simulink model "MODELODETURBINADERIOV10"  (R2017b)
settings: Solver=ode1  StartTime=0.0  StopTime=1  FixedStep=Ts  MaxStep=1e-6  MinStep=1e-7  RelTol=1e-4  AbsTol=1e-3
values from neighbouring files (symbols this model uses):
  A = pi()*((D/2)^2)    [MODELOHIDRO.m]    (also in MODELOHIDROV10.m; MODELOHIDROV2.m; MODELOHIDROV3.m; MODELOHIDROV4.m)
  B = 0    [MODELOHIDRO.m]    (also in MODELOHIDROV10.m; MODELOHIDROV2.m; MODELOHIDROV3.m; MODELOHIDROV4.m)
  beta = 0    [MODELOHIDRO.m]    (also in MODELOHIDROV10.m; MODELOHIDROV2.m; MODELOHIDROV3.m; MODELOHIDROV4.m)
  Cinv = 10e-6    (= 1e-05)    [MODELOHIDROV10.m]    (also in MODELOHIDROV4.m; MODELOHIDROV7.m; MODELOHIDROV8.m = 3e-06)
  den = 1000    [MODELOHIDRO.m]    (also in MODELOHIDROV10.m; MODELOHIDROV2.m; MODELOHIDROV3.m; MODELOHIDROV4.m)
  J = 16.1919e-4    (= 0.00161919)    [MODELOHIDROV10.m]    (also in MODELOHIDROV2.m = 100; MODELOHIDROV3.m = 10; MODELOHIDROV4.m; MODELOHIDROV7.m)
  K1Ic = 100    [MODELOHIDROV10.m]    (also in MODELOHIDROV4.m; MODELOHIDROV7.m; MODELOHIDROV8.m; stateStadeInv.m)
  K1Vo = 50    [MODELOHIDROV10.m]    (also in MODELOHIDROV4.m; MODELOHIDROV7.m; MODELOHIDROV8.m; stateStadeInv.m)
  K2Ic = 5    [MODELOHIDROV10.m]    (also in MODELOHIDROV4.m; MODELOHIDROV7.m; MODELOHIDROV8.m; stateStadeInv.m)
  K2Vo = 0.5    [MODELOHIDROV10.m]    (also in MODELOHIDROV4.m; MODELOHIDROV7.m; MODELOHIDROV8.m; stateStadeInv.m)
  Kb = 1.8    [MODELOHIDRO.m]    (also in MODELOHIDROV10.m = 6.2; MODELOHIDROV2.m; MODELOHIDROV3.m; MODELOHIDROV4.m = 0.027)
  Kp = 0.4    [MODELOHIDRO.m]    (also in MODELOHIDROV10.m = 5.6627; MODELOHIDROV2.m; MODELOHIDROV3.m; MODELOHIDROV4.m = 0.027)
  Linv = 25e-3    (= 0.025)    [MODELOHIDROV10.m]    (also in MODELOHIDROV4.m; MODELOHIDROV7.m; MODELOHIDROV8.m = 0.02345)
  r = D/2    (= 0.5)    [MODELOHIDRO.m]    (also in MODELOHIDROV10.m; MODELOHIDROV2.m; MODELOHIDROV3.m; MODELOHIDROV4.m)
  Ri = 0.6    [MODELOHIDRO.m]    (also in MODELOHIDROV10.m = 0.973; MODELOHIDROV2.m; MODELOHIDROV3.m; MODELOHIDROV4.m = 1)
  T_d = 0    [MODELOHIDRO.m]    (also in MODELOHIDROV10.m; MODELOHIDROV2.m; MODELOHIDROV3.m; MODELOHIDROV4.m)
  Vg = 150    [MODELOHIDROV10.m]    (also in MODELOHIDROV4.m; MODELOHIDROV7.m; MODELOHIDROV8.m)
undefined symbols (not defined in the file or in its folder): sigbuilder_block
libraries: powerlib_extras x3, simulink x2, powerlib_meascontrol x1
settings Model: ExtModeTrigMode=oneshot  ExtModeArmWhenConnect=off  ExtModeAutoUpdateStatusClock=off  Creator=Giroux/Sybille  LastModifiedBy=Hp 14
settings DataIOCC: SaveFinalState=on  SaveFormat=Structure  SignalLoggingSaveFormat=ModelDataLogs  SaveOutput=off  SaveTime=off  SignalLoggingName=sigsOut
settings OptimizationCC: BlockReduction=off  BooleanDataType=off  ExpressionDepthLimit=2147483647  InitFltsAndDblsToZero=on  LifeSpan=inf  BufferReusableBoundary=off
settings DebuggingCC: UnderspecifiedInitializationDetection=Classic  MergeDetectMultiDrivingBlocksExec=none  CheckExecutionContextPreStartOutputMsg=on  CheckExecutionContextRuntimeOutputMsg=on  SignalResolutionControl=TryResolveAllWithWarning  MultiTaskDSMMsg=warning  MultiTaskCondExecSysMsg=none  FcnCallInpInsideContextMsg=warning  UnconnectedLineMsg=none  BusObjectLabelMismatch=none  StateNameClashWarn=warning  SFUnexpectedBacktrackingDiag=warning  SFNoUnconditionalDefaultTransitionDiag=warning  SFExecutionAtInitializationDiag=none
settings HardwareCC: ProdBitPerPointer=32  ProdBitPerSizeT=32  ProdBitPerPtrDiffT=32  ProdLargestAtomicFloat=None  ProdIntDivRoundTo=Undefined  ProdEndianess=Unspecified  ProdWordSize=32  ProdHWDeviceType=32-bit Generic  TargetBitPerPointer=64  TargetBitPerSizeT=64  TargetBitPerPtrDiffT=64  TargetLongLongMode=on  TargetIntDivRoundTo=Zero  TargetEndianess=LittleEndian  TargetWordSize=64  TargetHWDeviceType=MATLAB Host  ProdEqTarget=off
settings ModelReferenceCC: PropagateSignalLabelsOutOfModel=off
settings CodeAppCC: StateflowObjectComments=on
settings GRTTargetCC: TargetLangStandard=C89/C90 (ANSI)  GeneratePreprocessorConditionals=Disable all  CombineOutputUpdateFcns=off  GRTInterface=on
settings ConfigComp: CovMetricSettings=dw  CovHtmlReporting=on  CovSaveCumulativeToWorkspaceVar=on  CovSaveSingleToWorkspaceVar=on  CovExternalEMLEnable=off
settings SimscapeCC: SimscapeNormalizeSystem=off

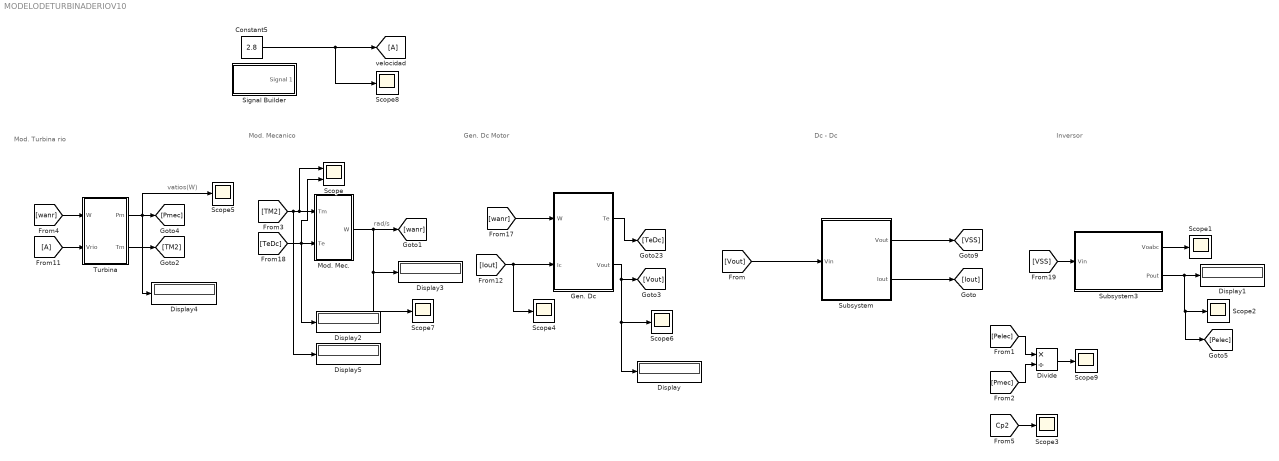
== system MODELODETURBINADERIOV10 ==
  note: vatios(W)
  note: rad/s
  note: Mod. Mecanico
  note: Gen. Dc Motor
  note: Mod. Turbina rio
  note: Inversor
  note: Dc - Dc
  Constant5 : Constant  Value=2.8
  Display{,1..5} (6 alike) : Display
  Divide : Product  Inputs=*/
  Gen. Dc : Subsystem
  Mod. Mec. : Subsystem
  Scope : Scope  NumInputPorts=2
  Scope{1..9} (9 alike) : Scope
  Signal Builder : Subsystem  Tag=STV Subsys  LoadFcn=sigbuilder_block('load');  StartFcn=sigbuilder_block('start');  StopFcn=sigbuilder_block('stop');  ClipboardFcn=sigbuilder_block('clipboard');  mask(Sigbuilder block){tuvar=[0:10]}
      mask help: Simulink:masks:SigbuilderBlock_MD
      mask init:
      | if ~strcmp(get_param(bdroot(gcbh),'SimulationStatus'),'stopped') tuvar = sigbuilder_block('maskInit'); end
      settings: CopyFcn=sigbuilder_block('copy');  DeleteFcn=sigbuilder_block('delete');  ModelCloseFcn=sigbuilder_block('modelClose');  PreSaveFcn=sigbuilder_block('preSave');  PauseFcn=sigbuilder_block('pause');  ContinueFcn=sigbuilder_block('continue');  NameChangeFcn=sigbuilder_block('namechange');  OpenFcn=sigbuilder_block('open',[437.25 153 550.5 359.25 ]);  CloseFcn=sigbuilder_block('close');
      mask Display: plot(0, 0, 100, 100,[2, 2, 32, 32, 2], [68, 8, 8, 68, 68],[32, 2], [38, 38], [32, 19, 2],[53, 60, 44], [32, 17, 17, 2],[16, 16, 31, 31]);txt = getActiveGroup(gcbh);text(2, 100, txt,'verticalAlignment', 'top');
  Subsystem : Subsystem
  Subsystem3 : Subsystem
  Turbina : Subsystem
  wires:
  [wanr] -> Gen. Dc/1(W)
  [TM2] -> Scope/1, Mod. Mec./1(Tm), Display5/1
  [wanr] -> Turbina/1(W)
  [TeDc] -> Display2/1, Scope/2, Mod. Mec./2(Te)
  Gen. Dc/1(Te) -> [TeDc]
  Turbina/1(Pm) -> [Pmec], Scope5/1, Display4/1
  Gen. Dc/2(Vout) -> [Vout], Scope6/1, Display/1
  Turbina/2(Tm) -> [TM2]
  [A] -> Turbina/2(Vrio)
  [Iout] -> Scope4/1, Gen. Dc/2(Ic)
  [VSS] -> Subsystem3/1(Vin)
  Subsystem3/1("Voabc ") -> Scope1/1
  Subsystem/1(Vout) -> [VSS]
  Subsystem/2(Iout) -> [Iout]
  [Vout] -> Subsystem/1(Vin)
  Subsystem3/2(Pout) -> Scope2/1, [Pelec], Display1/1
  [Pelec] -> Divide/1
  [Pmec] -> Divide/2
  Divide/1 -> Scope9/1
  [Cp2] -> Scope3/1
  Mod. Mec./1(W) -> Scope7/1, Display3/1, [wanr]
  Constant5/1 -> [A], Scope8/1

== system MODELODETURBINADERIOV10/Gen. Dc ==
  note: Calculo del par electrico con la corriente en la carga
  note: Se emplean parametro de un motor dc para 18.5Kw debido a que fueron con los que mejor trabajo
  W : Inport
  Ic : Inport  Port=2
  Motor iman. : Subsystem
  Par elec. : Subsystem
  Te : Outport
  Vout : Outport  Port=2
  wires:
  Motor iman./1(Out1) -> Vout/1
  Par elec./1(Te) -> Te/1
  W/1 -> Motor iman./2(W)
  Ic/1 -> Par elec./1(Ic), Motor iman./1(I)

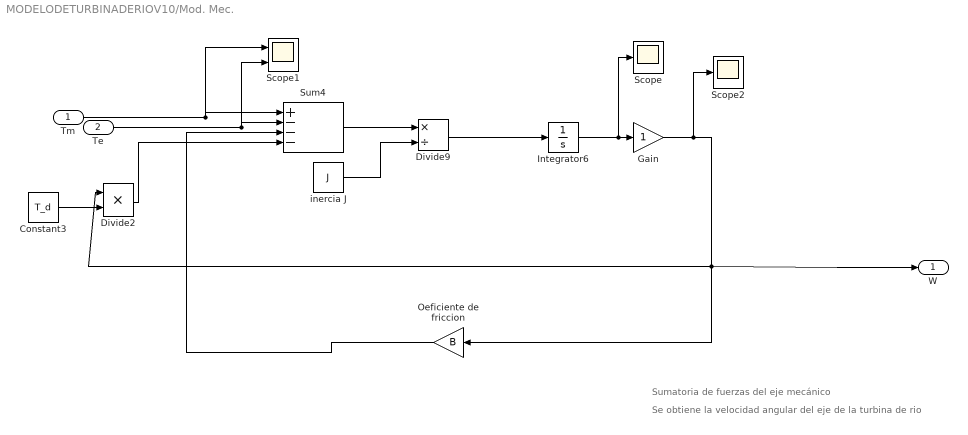
== system MODELODETURBINADERIOV10/Mod. Mec. ==
  note: Se obtiene la velocidad angular del eje de la turbina de rio
  note: Sumatoria de fuerzas del eje mecánico
  Tm : Inport
  Te : Inport  Port=2
  Constant3 : Constant  Value=T_d
  Divide2 : Product  Inputs=**
  Divide9 : Product  Inputs=*/
  Gain : Gain
  Integrator6 : Integrator  InitialCondition=10
  Oeficiente de friccion : Gain  Gain=B
  Scope : Scope
  Scope1 : Scope  NumInputPorts=2
  Scope2 : Scope
  Sum4 : Sum  Inputs=|+---
  inercia J : Constant  Value=J
  W : Outport
  wires:
  inercia J/1 -> Divide9/2
  Constant3/1 -> Divide2/2
  Divide2/1 -> Sum4/4
  Oeficiente de friccion/1 -> Sum4/3
  Sum4/1 -> Divide9/1
  Tm/1 -> Scope1/1, Sum4/1
  Te/1 -> Scope1/2, Sum4/2
  Divide9/1 -> Integrator6/1
  Integrator6/1 -> Scope/1, Gain/1
  Gain/1 -> Scope2/1, Oeficiente de friccion/1, W/1, Divide2/1

== system MODELODETURBINADERIOV10/Signal Builder ==
  Demux : Demux  Tag=STV Demux  Outputs=1
  FromWs : FromWorkspace  Tag=STV FromWs  VariableName=tuvar  SampleTime=0
      SigBuilderData=|
      | common.afterFinalStr = 'Extrapolate'
      | common.sampleTime = 0
      | dataSet.timeRange = [0 1]
      | dataSet.name = 'Group 1'
      | sbobj.Groups.Name = 'Group 1'
      | sbobj.Groups.Signals.Name = 'Signal 1'
      | sbobj.Groups.Signals.XData = [0 0.32 0.32 1]
      | sbobj.Groups.Signals.YData = [2.6 2.6 2.8 2.8]
      | sbobj.Groups.TimeRange = [0 1]
  Signal 1 : Outport  Tag=STV Outport
  wires:
  Demux/1 -> Signal 1/1
  FromWs/1 -> Demux/1

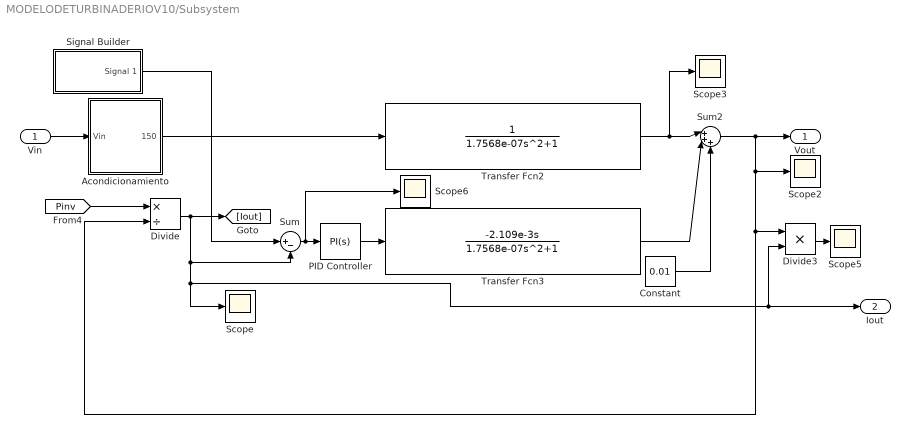
== system MODELODETURBINADERIOV10/Subsystem ==
  Vin : Inport
  Acondicionamiento : Subsystem
  Constant : Constant  Value=0.01
  Divide : Product  Inputs=*/
  Divide3 : Product  Inputs=**
  PID Controller : simulink/Continuous/PID Controller  Controller=PI  TimeDomain=Continuous-time  SampleTime=-1  IntegratorMethod=Forward Euler  FilterMethod=Forward Euler  Form=Parallel  UseFilter=on  ControllerParametersSource=internal  P=30  I=55  D=0  N=100  InitialConditionSource=internal  InitialConditionForIntegrator=0  InitialConditionForFilter=0  ExternalReset=none  LimitOutput=off  UpperSaturationLimit=inf  LowerSaturationLimit=-inf  LinearizeAsGain=on  AntiWindupMode=none  Kb=1  TrackingMode=off  Kt=1  PParamMin=[]  PParamMax=[]  IParamMin=[]  IParamMax=[]  DParamMin=[]  DParamMax=[]  NParamMin=[]  NParamMax=[]  KbParamMin=[]  KbParamMax=[]  KtParamMin=[]  KtParamMax=[]  POutMin=[]  POutMax=[]  IOutMin=[]  IOutMax=[]  DOutMin=[]  DOutMax=[]  NOutMin=[]  NOutMax=[]  KbOutMin=[]  KbOutMax=[]  KtOutMin=[]  KtOutMax=[]  IntegratorOutMin=[]  IntegratorOutMax=[]  FilterOutMin=[]  FilterOutMax=[]  SumOutMin=[]  SumOutMax=[]  SumI1OutMin=[]  SumI1OutMax=[]  SumI2OutMin=[]  SumI2OutMax=[]  SumI3OutMin=[]  SumI3OutMax=[]  SumDOutMin=[]  SumDOutMax=[]  SaturationOutMin=[]  SaturationOutMax=[]  IntegratorContinuousStateAttributes=''  IntegratorStateMustResolveToSignalObject=off  IntegratorRTWStateStorageClass=Auto  FilterContinuousStateAttributes=''  FilterStateMustResolveToSignalObject=off  FilterRTWStateStorageClass=Auto  DifferentiatorICPrevScaledInput=0  DifferentiatorOutMin=[]  DifferentiatorOutMax=[]  InitialConditionSetting=State (most efficient)  FilterDiffOutCoefMin=[]  FilterDiffOutCoefMax=[]  SumDenOutMin=[]  SumDenOutMax=[]  SumNumOutMin=[]  SumNumOutMax=[]  ReciprocalOutMin=[]  ReciprocalOutMax=[]  DivideOutMin=[]  DivideOutMax=[]  TunerSelectOption=Transfer Function Based (PID Tuner App)
  Scope{,2..3,5..6} (5 alike) : Scope
  Signal Builder : Subsystem  Tag=STV Subsys  LoadFcn=sigbuilder_block('load');  StartFcn=sigbuilder_block('start');  StopFcn=sigbuilder_block('stop');  ClipboardFcn=sigbuilder_block('clipboard');  mask(Sigbuilder block){tuvar=[0:10]}
      mask help: Simulink:masks:SigbuilderBlock_MD
      mask init:
      | if ~strcmp(get_param(bdroot(gcbh),'SimulationStatus'),'stopped') tuvar = sigbuilder_block('maskInit'); end
      settings: CopyFcn=sigbuilder_block('copy');  DeleteFcn=sigbuilder_block('delete');  ModelCloseFcn=sigbuilder_block('modelClose');  PreSaveFcn=sigbuilder_block('preSave');  PauseFcn=sigbuilder_block('pause');  ContinueFcn=sigbuilder_block('continue');  NameChangeFcn=sigbuilder_block('namechange');  OpenFcn=sigbuilder_block('open',[437.25 153 550.5 359.25 ]);  CloseFcn=sigbuilder_block('close');
      mask Display: plot(0, 0, 100, 100,[2, 2, 32, 32, 2], [68, 8, 8, 68, 68],[32, 2], [38, 38], [32, 19, 2],[53, 60, 44], [32, 17, 17, 2],[16, 16, 31, 31]);txt = getActiveGroup(gcbh);text(2, 100, txt,'verticalAlignment', 'top');
  Sum : Sum  Inputs=|+-
  Sum2 : Sum  Inputs=|+++
  Transfer Fcn2 : TransferFcn  Denominator=[1.7568e-07 0 1]
  Transfer Fcn3 : TransferFcn  Numerator=[-2.109e-3 0]  Denominator=[1.7568e-07 0 1]
  Vout : Outport
  Iout : Outport  Port=2
  wires:
  Transfer Fcn3/1 -> Sum2/2
  Transfer Fcn2/1 -> Scope3/1, Sum2/1
  Vin/1 -> Acondicionamiento/1(Vin)
  [Pinv] -> Divide/1
  Divide/1 -> Sum/2, Divide3/2, Iout/1, Scope/1, [Iout]
  Constant/1 -> Sum2/3
  Sum2/1 -> Divide/2, Divide3/1, Scope2/1, Vout/1
  Divide3/1 -> Scope5/1
  Acondicionamiento/1(150) -> Transfer Fcn2/1
  PID Controller/1 -> Transfer Fcn3/1
  Sum/1 -> Scope6/1, PID Controller/1
  Signal Builder/1(Signal 1) -> Sum/1

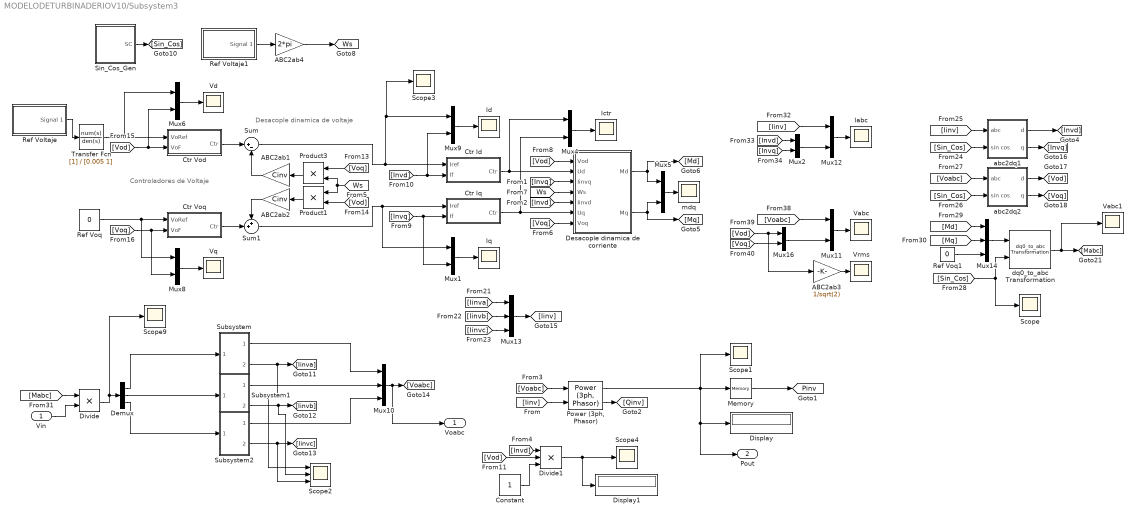
== system MODELODETURBINADERIOV10/Subsystem3 ==
  note: Desacople dinamica de voltaje
  note: Controladores de Voltaje
  Vin : Inport
  ABC2ab1 : Gain  Gain=Cinv  SaturateOnIntegerOverflow=on  OutDataTypeStr=Inherit: Same as input  ParamDataTypeStr=Inherit: Same as input
  ABC2ab2 : Gain  Gain=Cinv  SaturateOnIntegerOverflow=on  OutDataTypeStr=Inherit: Same as input  ParamDataTypeStr=Inherit: Same as input
  ABC2ab3 : Gain  Gain=1/sqrt(2)  SaturateOnIntegerOverflow=on  OutDataTypeStr=Inherit: Same as input  ParamDataTypeStr=Inherit: Same as input
  ABC2ab4 : Gain  Gain=2*pi  SaturateOnIntegerOverflow=on  OutDataTypeStr=Inherit: Same as input  ParamDataTypeStr=Inherit: Same as input
  Constant : Constant
  Ctr Id : Subsystem
  Ctr Iq : Subsystem
  Ctr Vod : Subsystem
  Ctr Voq : Subsystem
  Demux : Demux  Outputs=3
  Desacople dinamica de corriente : Subsystem
  Display : Display
  Display1 : Display
  Divide : Product  Inputs=**
  Divide1 : Product  Inputs=***
  Iabc : Scope
  Ictr : Scope
  Id : Scope
  Iq : Scope
  Memory : Memory
  Mux{1..2,4..6,8..9,11..12,16} (10 alike) : Mux  Inputs=2
  Mux10 : Mux  Inputs=3
  Mux13 : Mux  Inputs=3
  Mux14 : Mux  Inputs=3
  "Power (3ph, Phasor)" : powerlib_meascontrol/Measurements/Power (3ph, Phasor)
      settings: SourceProductName=Simscape Power Systems  SourceProductBaseCode=PS
  Product1 : Product  OutDataTypeStr=double  RndMeth=Zero
  Product3 : Product  OutDataTypeStr=double  RndMeth=Zero
  Ref Voltaje : Subsystem  Tag=STV Subsys  LoadFcn=sigbuilder_block('load');  StartFcn=sigbuilder_block('start');  StopFcn=sigbuilder_block('stop');  ClipboardFcn=sigbuilder_block('clipboard');  mask(Sigbuilder block){tuvar=[0:10]}
      mask help: Sigbuilder GUI
      mask init:
      | if ~strcmp(get_param(bdroot(gcbh),'SimulationStatus'),'stopped') tuvar = sigbuilder_block('maskInit'); end
      settings: CopyFcn=sigbuilder_block('copy');  DeleteFcn=sigbuilder_block('delete');  ModelCloseFcn=sigbuilder_block('modelClose');  PreSaveFcn=sigbuilder_block('preSave');  PauseFcn=sigbuilder_block('pause')  ContinueFcn=sigbuilder_block('continue')  NameChangeFcn=sigbuilder_block('namechange');  OpenFcn=sigbuilder_block('open',[437.25 117 550.5 399 ]);  CloseFcn=sigbuilder_block('close');
      mask Display: plot(0, 0, 100, 100,[2, 2, 32, 32, 2], [68, 8, 8, 68, 68],[32, 2], [38, 38], [32, 19, 2],[53, 60, 44], [32, 17, 17, 2],[16, 16, 31, 31]);txt = getActiveGroup(gcbh);text(2, 100, txt,'verticalAlignment', 'top');
  Ref Voltaje1 : Subsystem  Tag=STV Subsys  LoadFcn=sigbuilder_block('load');  StartFcn=sigbuilder_block('start');  StopFcn=sigbuilder_block('stop');  ClipboardFcn=sigbuilder_block('clipboard');  mask(Sigbuilder block){tuvar=[0:10]}
      mask help: Sigbuilder GUI
      mask init:
      | if ~strcmp(get_param(bdroot(gcbh),'SimulationStatus'),'stopped') tuvar = sigbuilder_block('maskInit'); end
      settings: CopyFcn=sigbuilder_block('copy');  DeleteFcn=sigbuilder_block('delete');  ModelCloseFcn=sigbuilder_block('modelClose');  PreSaveFcn=sigbuilder_block('preSave');  PauseFcn=sigbuilder_block('pause')  ContinueFcn=sigbuilder_block('continue')  NameChangeFcn=sigbuilder_block('namechange');  OpenFcn=sigbuilder_block('open',[437.25 117 550.5 399 ]);  CloseFcn=sigbuilder_block('close');
      mask Display: plot(0, 0, 100, 100,[2, 2, 32, 32, 2], [68, 8, 8, 68, 68],[32, 2], [38, 38], [32, 19, 2],[53, 60, 44], [32, 17, 17, 2],[16, 16, 31, 31]);txt = getActiveGroup(gcbh);text(2, 100, txt,'verticalAlignment', 'top');
  Ref Voq : Constant  Value=0
  Ref Voq1 : Constant  Value=0
  Scope{,1,3..4,9} (5 alike) : Scope
  Scope2 : Scope  NumInputPorts=3
  Sin_Cos_Gen : Subsystem
  Subsystem : Subsystem
  Subsystem1 : Subsystem
  Subsystem2 : Subsystem
  Sum : Sum  Inputs=|+-
  Sum1 : Sum  Inputs=++|
  Transfer Fcn : TransferFcn  Denominator=[0.005 1]
  Vabc : Scope
  Vabc1 : Scope
  Vd : Scope
  Vq : Scope
  Vrms : Scope
  abc2dq1 : Subsystem
  abc2dq2 : Subsystem
  dq0_to_abc Transformation : powerlib_extras/Measurements/dq0_to_abc Transformation
  mdq : Scope
  "Voabc " : Outport
  Pout : Outport  Port=2
  tag scope: Pinv=global, Ws=global
  wires:
  Demux/2 -> Subsystem1/1(Vin)
  Subsystem2/2(Iout) -> Scope2/3, [Iinvc]
  Subsystem1/1(Vout) -> Mux10/2
  Subsystem/2(Iout) -> Scope2/1, [Iinva]
  Mux9/1 -> Id/1
  [Vod] -> Desacople dinamica de corriente/1(Vod)
  Ctr Id/1(Ctr) -> Desacople dinamica de corriente/2(Ud), Mux4/1
  [Invd] -> Desacople dinamica de corriente/5(Iinvd)
  [Invq] -> Desacople dinamica de corriente/3(Iinvq)
  Mux4/1 -> Ictr/1
  Mux5/1 -> mdq/1
  Product1/1 -> ABC2ab2/1
  [Invq] -> Ctr Iq/2(If), Mux1/2
  [Invd] -> Ctr Id/2(If), Mux9/2
  [Voq] -> Desacople dinamica de corriente/7(Voq)
  ABC2ab4/1 -> [Ws]
  [Ws] -> Desacople dinamica de corriente/4(Ws)
  Sum1/1 -> Ctr Iq/1(Iref), Mux1/1
  Ctr Iq/1(Ctr) -> Desacople dinamica de corriente/6(Uq), Mux4/2
  Mux1/1 -> Iq/1
  [Ws] -> Product3/2, Product1/1
  Sum/1 -> Ctr Id/1(Iref), Scope3/1, Mux9/1
  ABC2ab1/1 -> Sum/2
  Product3/1 -> ABC2ab1/1
  [Voq] -> Product3/1
  Mux6/1 -> Vd/1
  [Vod] -> Mux6/2, Ctr Vod/2(VoF)
  Ctr Voq/1(Ctr) -> Sum1/2
  ABC2ab2/1 -> Sum1/1
  [Vod] -> Product1/2
  Ctr Vod/1(Ctr) -> Sum/1
  Ref Voq/1 -> Mux8/1, Ctr Voq/1(VoRef)
  Ref Voltaje/1(Signal 1) -> Transfer Fcn/1
  [Voq] -> Mux8/2, Ctr Voq/2(VoF)
  Mux8/1 -> Vq/1
  [Iinva] -> Mux13/1
  Mux13/1 -> [Iinv]
  Mux12/1 -> Iabc/1
  [Iinv] -> abc2dq1/1(abc)
  [Iinvb] -> Mux13/2
  [Sin_Cos] -> abc2dq1/2(sin cos)
  Mux11/1 -> Vabc/1
  [Iinvc] -> Mux13/3
  [Iinv] -> Mux12/1
  [Voabc] -> abc2dq2/1(abc)
  [Vod] -> Mux16/1, ABC2ab3/1
  ABC2ab3/1 -> Vrms/1
  Sin_Cos_Gen/1(SC) -> [Sin_Cos]
  Ref Voq1/1 -> Mux14/3
  [Md] -> Mux14/1
  Desacople dinamica de corriente/2(Mq) -> Mux5/2, [Mq]
  abc2dq2/2(q) -> [Voq]
  [Sin_Cos] -> abc2dq2/2(sin cos)
  [Mq] -> Mux14/2
  dq0_to_abc Transformation/1 -> [Mabc], Vabc1/1
  abc2dq1/2(q) -> [Invq]
  abc2dq2/1(d) -> [Vod]
  [Sin_Cos] -> Scope/1, dq0_to_abc Transformation/2
  [Invd] -> Mux2/1
  Desacople dinamica de corriente/1(Md) -> Mux5/1, [Md]
  [Voabc] -> Mux11/1
  Mux2/1 -> Mux12/2
  [Invq] -> Mux2/2
  [Voq] -> Mux16/2
  Mux16/1 -> Mux11/2
  Mux14/1 -> dq0_to_abc Transformation/1
  Ref Voltaje1/1(Signal 1) -> ABC2ab4/1
  Transfer Fcn/1 -> Mux6/1, Ctr Vod/1(VoRef)
  Subsystem/1(Vout) -> Mux10/1
  Demux/3 -> Subsystem2/1(Vin)
  Demux/1 -> Subsystem/1(Vin)
  Mux10/1 -> "Voabc "/1, [Voabc]
  Subsystem1/2(Iout) -> Scope2/2, [Iinvb]
  [Mabc] -> Divide/1
  Divide/1 -> Scope9/1, Demux/1
  Subsystem2/1(Vout) -> Mux10/3
  [Iinv] -> "Power (3ph, Phasor)"/2
  [Voabc] -> "Power (3ph, Phasor)"/1
  "Power (3ph, Phasor)"/1 -> Pout/1, Display/1, Scope1/1, Memory/1
  "Power (3ph, Phasor)"/2 -> [Qinv]
  Memory/1 -> [Pinv]
  Vin/1 -> Divide/2
  abc2dq1/1(d) -> [Invd]
  Constant/1 -> Divide1/3
  [Invd] -> Divide1/1
  [Vod] -> Divide1/2
  Divide1/1 -> Display1/1, Scope4/1

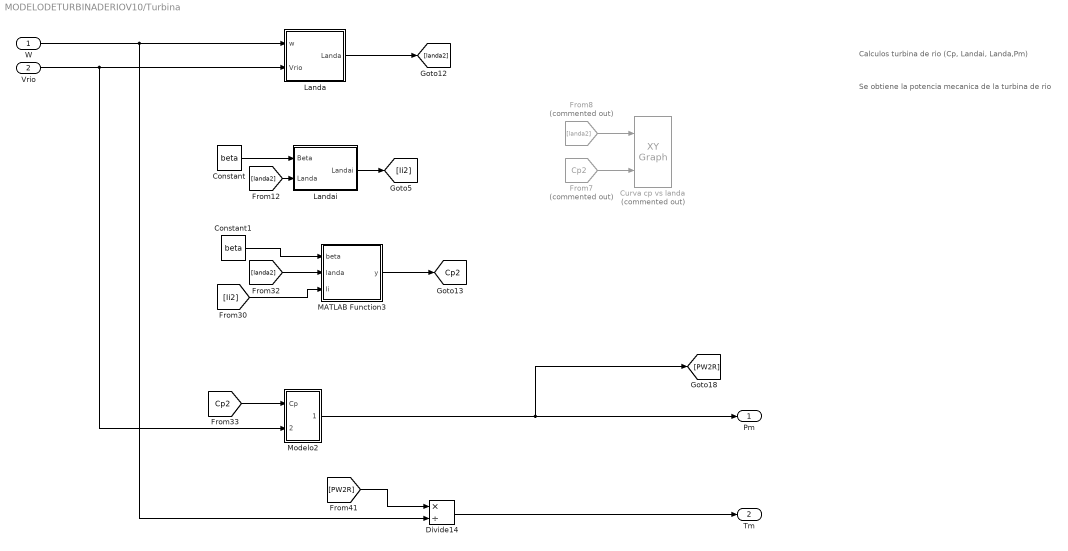
== system MODELODETURBINADERIOV10/Turbina ==
  note: Calculos turbina de rio (Cp, Landai, Landa,Pm)
  note: Se obtiene la potencia mecanica de la turbina de rio
  W : Inport
  Vrio : Inport  Port=2
  Constant : Constant  Value=beta
  Constant1 : Constant  Value=beta
  Curva cp vs landa : simulink/Sinks/XY Graph  Commented=on  xmin=1  xmax=20  ymin=0  ymax=0.56  st=0.1
  Divide14 : Product  Inputs=*/
  From7 : From  Commented=on  GotoTag=Cp2
  From8 : From  Commented=on  GotoTag=landa2
  Landa : Subsystem
  Landai : Subsystem
  MATLAB Function3 : MATLAB Function  TreatAsAtomicUnit=on
  Modelo2 : Subsystem
  Pm : Outport
  Tm : Outport  Port=2
  tag scope: Cp2=global
  wires:
  Constant1/1 -> MATLAB Function3/1(beta)
  Divide14/1 -> Tm/1
  [Ii2] -> MATLAB Function3/3(Ii)
  [Cp2] -> Modelo2/1(Cp)
  [PW2R] -> Divide14/1
  W/1 -> Divide14/2, Landa/1(w)
  [landa2] -> MATLAB Function3/2(landa)
  Vrio/1 -> Modelo2/2(Vrio), Landa/2(Vrio)
  Landa/1(Landa) -> [landa2]
  MATLAB Function3/1(y) -> [Cp2]
  From8/1 -> Curva cp vs landa/1
  Constant/1 -> Landai/1(Beta)
  [landa2] -> Landai/2(Landa)
  Modelo2/1(Pm) -> [PW2R], Pm/1
  Landai/1(Landai) -> [Ii2]
  From7/1 -> Curva cp vs landa/2

== system MODELODETURBINADERIOV10/Gen. Dc/Motor iman. ==
  note: Se obtiene la tension del generador a partir de una velocidad angular
  note: y una corriente retroalimentada del conversor dc-dc
  I : Inport
  W : Inport  Port=2
  Constant1 : Constant  Value=Kb
  Constant2 : Constant  Value=Ri
  Divide6 : Product  Inputs=**  SaturateOnIntegerOverflow=on  RndMeth=Zero
  Divide7 : Product  Inputs=**  SaturateOnIntegerOverflow=on  RndMeth=Zero
  Sum1 : Sum
  Out1 : Outport
  wires:
  Divide7/1 -> Sum1/2
  Divide6/1 -> Sum1/1
  I/1 -> Divide7/2
  Constant2/1 -> Divide7/1
  Constant1/1 -> Divide6/1
  W/1 -> Divide6/2
  Sum1/1 -> Out1/1

== system MODELODETURBINADERIOV10/Gen. Dc/Par elec. ==
  Ic : Inport
  Constant2 : Constant  Value=Kp
  Divide2 : Product  Inputs=**
  Te : Outport
  wires:
  Ic/1 -> Divide2/1
  Constant2/1 -> Divide2/2
  Divide2/1 -> Te/1

== system MODELODETURBINADERIOV10/Subsystem/Acondicionamiento ==
  note: Se garantiza una entrada fija a 150, pero si la tension de entrada desciende
      | se deja su valor original y se calcula con ello el ciclo Duty
  Vin : Inport
  Constant1 : Constant  Value=300
  Divide : Product  Inputs=**
  Divide1 : Product  Inputs=*/
  Saturation : Saturate  UpperLimit=1  LowerLimit=0
  150 : Outport
  wires:
  Divide1/1 -> Saturation/1
  Divide/1 -> 150/1
  Saturation/1 -> Divide/2
  Constant1/1 -> Divide1/1
  Vin/1 -> Divide/1, Divide1/2

== system MODELODETURBINADERIOV10/Subsystem/Signal Builder ==
  Demux : Demux  Tag=STV Demux  Outputs=1
  FromWs : FromWorkspace  Tag=STV FromWs  VariableName=tuvar  SampleTime=0
      SigBuilderData=|
      | common.afterFinalStr = 'Extrapolate'
      | common.sampleTime = 0
      | dataSet.timeRange = [0 1]
      | dataSet.name = 'Group 1'
      | sbobj.Groups.Name = 'Group 1'
      | sbobj.Groups.Signals.Name = 'Signal 1'
      | sbobj.Groups.Signals.XData = [0 1]
      | sbobj.Groups.Signals.YData = [1 1]
      | sbobj.Groups.TimeRange = [0 1]
  Signal 1 : Outport  Tag=STV Outport
  wires:
  Demux/1 -> Signal 1/1
  FromWs/1 -> Demux/1

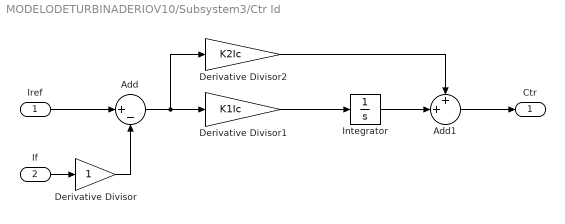
== system MODELODETURBINADERIOV10/Subsystem3/Ctr Id ==
  Iref : Inport
  If : Inport  Port=2
  Add : Sum  Inputs=|+-
  Add1 : Sum  Inputs=++|
  Derivative Divisor : Gain  SaturateOnIntegerOverflow=on  OutDataTypeStr=Inherit: Same as input  ParamDataTypeStr=Inherit: Same as input
  Derivative Divisor1 : Gain  Gain=K1Ic  SaturateOnIntegerOverflow=on  OutDataTypeStr=Inherit: Same as input  ParamDataTypeStr=Inherit: Same as input
  Derivative Divisor2 : Gain  Gain=K2Ic  SaturateOnIntegerOverflow=on  OutDataTypeStr=Inherit: Same as input  ParamDataTypeStr=Inherit: Same as input
  Integrator : Integrator
  Ctr : Outport
  wires:
  If/1 -> Derivative Divisor/1
  Derivative Divisor/1 -> Add/2
  Add/1 -> Derivative Divisor1/1, Derivative Divisor2/1
  Derivative Divisor1/1 -> Integrator/1
  Integrator/1 -> Add1/2
  Derivative Divisor2/1 -> Add1/1
  Add1/1 -> Ctr/1
  Iref/1 -> Add/1

== system MODELODETURBINADERIOV10/Subsystem3/Ctr Iq ==
  Iref : Inport
  If : Inport  Port=2
  Add : Sum  Inputs=|+-
  Add1 : Sum  Inputs=++|
  Derivative Divisor : Gain  SaturateOnIntegerOverflow=on  OutDataTypeStr=Inherit: Same as input  ParamDataTypeStr=Inherit: Same as input
  Derivative Divisor1 : Gain  Gain=K1Ic  SaturateOnIntegerOverflow=on  OutDataTypeStr=Inherit: Same as input  ParamDataTypeStr=Inherit: Same as input
  Derivative Divisor2 : Gain  Gain=K2Ic  SaturateOnIntegerOverflow=on  OutDataTypeStr=Inherit: Same as input  ParamDataTypeStr=Inherit: Same as input
  Integrator : Integrator
  Ctr : Outport
  wires:
  Iref/1 -> Add/1
  Add1/1 -> Ctr/1
  Derivative Divisor2/1 -> Add1/1
  Integrator/1 -> Add1/2
  Derivative Divisor1/1 -> Integrator/1
  Add/1 -> Derivative Divisor2/1, Derivative Divisor1/1
  Derivative Divisor/1 -> Add/2
  If/1 -> Derivative Divisor/1

== system MODELODETURBINADERIOV10/Subsystem3/Ctr Vod ==
  VoRef : Inport
  VoF : Inport  Port=2
  Add : Sum  Inputs=|+-
  Add1 : Sum  Inputs=++|
  Derivative Divisor : Gain  SaturateOnIntegerOverflow=on  OutDataTypeStr=Inherit: Same as input  ParamDataTypeStr=Inherit: Same as input
  Derivative Divisor1 : Gain  Gain=K1Vo  SaturateOnIntegerOverflow=on  OutDataTypeStr=Inherit: Same as input  ParamDataTypeStr=Inherit: Same as input
  Derivative Divisor2 : Gain  Gain=K2Vo  SaturateOnIntegerOverflow=on  OutDataTypeStr=Inherit: Same as input  ParamDataTypeStr=Inherit: Same as input
  Integrator : Integrator
  Ctr : Outport
  wires:
  VoRef/1 -> Add/1
  Derivative Divisor2/1 -> Add1/1
  Integrator/1 -> Add1/2
  Derivative Divisor1/1 -> Integrator/1
  Add/1 -> Derivative Divisor2/1, Derivative Divisor1/1
  Derivative Divisor/1 -> Add/2
  VoF/1 -> Derivative Divisor/1
  Add1/1 -> Ctr/1

== system MODELODETURBINADERIOV10/Subsystem3/Ctr Voq ==
  VoRef : Inport
  VoF : Inport  Port=2
  Add : Sum  Inputs=|+-
  Add1 : Sum  Inputs=++|
  Derivative Divisor : Gain  SaturateOnIntegerOverflow=on  OutDataTypeStr=Inherit: Same as input  ParamDataTypeStr=Inherit: Same as input
  Derivative Divisor1 : Gain  Gain=K1Vo  SaturateOnIntegerOverflow=on  OutDataTypeStr=Inherit: Same as input  ParamDataTypeStr=Inherit: Same as input
  Derivative Divisor2 : Gain  Gain=K2Vo  SaturateOnIntegerOverflow=on  OutDataTypeStr=Inherit: Same as input  ParamDataTypeStr=Inherit: Same as input
  Integrator : Integrator
  Ctr : Outport
  wires:
  Add1/1 -> Ctr/1
  VoF/1 -> Derivative Divisor/1
  Derivative Divisor/1 -> Add/2
  Add/1 -> Derivative Divisor1/1, Derivative Divisor2/1
  Derivative Divisor1/1 -> Integrator/1
  Integrator/1 -> Add1/2
  Derivative Divisor2/1 -> Add1/1
  VoRef/1 -> Add/1

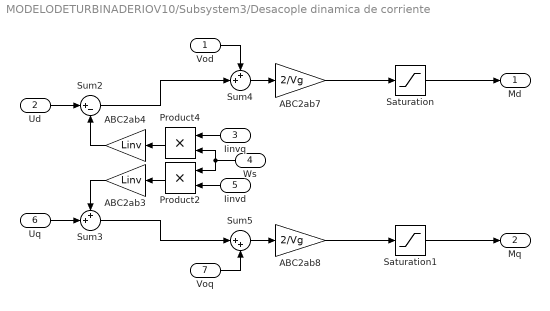
== system MODELODETURBINADERIOV10/Subsystem3/Desacople dinamica de corriente ==
  Vod : Inport
  Ud : Inport  Port=2
  Iinvq : Inport  Port=3
  Ws : Inport  Port=4
  Iinvd : Inport  Port=5
  Uq : Inport  Port=6
  Voq : Inport  Port=7
  ABC2ab3 : Gain  Gain=Linv  SaturateOnIntegerOverflow=on  OutDataTypeStr=Inherit: Same as input  ParamDataTypeStr=Inherit: Same as input
  ABC2ab4 : Gain  Gain=Linv  SaturateOnIntegerOverflow=on  OutDataTypeStr=Inherit: Same as input  ParamDataTypeStr=Inherit: Same as input
  ABC2ab7 : Gain  Gain=2/Vg  SaturateOnIntegerOverflow=on  OutDataTypeStr=Inherit: Same as input  ParamDataTypeStr=Inherit: Same as input
  ABC2ab8 : Gain  Gain=2/Vg  SaturateOnIntegerOverflow=on  OutDataTypeStr=Inherit: Same as input  ParamDataTypeStr=Inherit: Same as input
  Product2 : Product  OutDataTypeStr=double  RndMeth=Zero
  Product4 : Product  OutDataTypeStr=double  RndMeth=Zero
  Saturation : Saturate  UpperLimit=1  LowerLimit=-1
  Saturation1 : Saturate  UpperLimit=1  LowerLimit=-1
  Sum2 : Sum  Inputs=|+-
  Sum3 : Sum  Inputs=++|
  Sum4 : Sum  Inputs=++|
  Sum5 : Sum  Inputs=|++
  Md : Outport
  Mq : Outport  Port=2
  wires:
  Product4/1 -> ABC2ab4/1
  Product2/1 -> ABC2ab3/1
  Ws/1 -> Product4/2, Product2/1
  ABC2ab3/1 -> Sum3/1
  ABC2ab4/1 -> Sum2/2
  Vod/1 -> Sum4/1
  Iinvq/1 -> Product4/1
  Iinvd/1 -> Product2/2
  Voq/1 -> Sum5/2
  ABC2ab7/1 -> Saturation/1
  ABC2ab8/1 -> Saturation1/1
  Sum4/1 -> ABC2ab7/1
  Sum5/1 -> ABC2ab8/1
  Sum2/1 -> Sum4/2
  Sum3/1 -> Sum5/1
  Ud/1 -> Sum2/1
  Uq/1 -> Sum3/2
  Saturation/1 -> Md/1
  Saturation1/1 -> Mq/1

== system MODELODETURBINADERIOV10/Subsystem3/Ref Voltaje ==
  Demux : Demux  Tag=STV Demux  Outputs=1
  FromWs : FromWorkspace  Tag=STV FromWs  VariableName=tuvar  SampleTime=0
      SigBuilderData=|
      | common.afterFinalStr = 'Extrapolate'
      | common.sampleTime = 0
      | dataSet.timeRange = [0 0.8]
      | dataSet.name = 'Group 1'
      | sbobj.Name = 'Signal Builder'
      | sbobj.Groups.Name = 'Group 1'
      | sbobj.Groups.Signals.Name = 'Signal 1'
      | sbobj.Groups.Signals.XData = [0 0.025 0.8]
      | sbobj.Groups.Signals.YData = [-43.5 220 220]
      | sbobj.Groups.TimeRange = [0 0.8]
  Signal 1 : Outport  Tag=STV Outport
  wires:
  Demux/1 -> Signal 1/1
  FromWs/1 -> Demux/1

== system MODELODETURBINADERIOV10/Subsystem3/Ref Voltaje1 ==
  Demux : Demux  Tag=STV Demux  Outputs=1
  FromWs : FromWorkspace  Tag=STV FromWs  VariableName=tuvar  SampleTime=0
      SigBuilderData=|
      | common.afterFinalStr = 'Extrapolate'
      | common.sampleTime = 0
      | dataSet.timeRange = [0 1]
      | dataSet.name = 'Group 1'
      | sbobj.Name = 'Signal Builder'
      | sbobj.Groups.Name = 'Group 1'
      | sbobj.Groups.Signals.Name = 'Signal 1'
      | sbobj.Groups.Signals.XData = [0 0.025 0.025 0.5 1]
      | sbobj.Groups.Signals.YData = [1 57.5 60 60 60]
      | sbobj.Groups.TimeRange = [0 1]
  Signal 1 : Outport  Tag=STV Outport
  wires:
  FromWs/1 -> Demux/1
  Demux/1 -> Signal 1/1

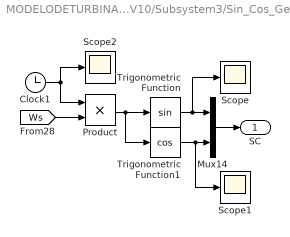
== system MODELODETURBINADERIOV10/Subsystem3/Sin_Cos_Gen ==
  Clock1 : Clock
  Mux14 : Mux  Inputs=2
  Product : Product  RndMeth=Zero
  Scope : Scope
  Scope1 : Scope
  Scope2 : Scope
  Trigonometric Function : Trigonometry
  Trigonometric Function1 : Trigonometry  Operator=cos
  SC : Outport
  wires:
  Product/1 -> Trigonometric Function/1, Trigonometric Function1/1
  Clock1/1 -> Scope2/1, Product/1
  [Ws] -> Product/2
  Trigonometric Function/1 -> Scope/1, Mux14/1
  Trigonometric Function1/1 -> Scope1/1, Mux14/2
  Mux14/1 -> SC/1

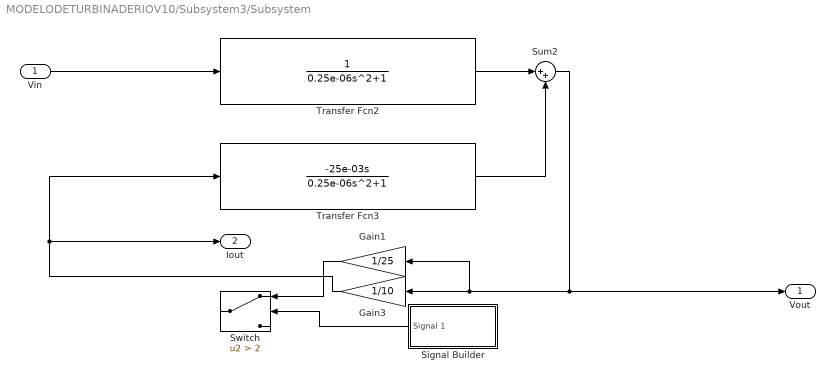
== system MODELODETURBINADERIOV10/Subsystem3/Subsystem ==
  Vin : Inport
  Gain1 : Gain  Gain=1/25
  Gain3 : Gain  Gain=1/10
  Signal Builder : Subsystem  Tag=STV Subsys  LoadFcn=sigbuilder_block('load');  StartFcn=sigbuilder_block('start');  StopFcn=sigbuilder_block('stop');  ClipboardFcn=sigbuilder_block('clipboard');  mask(Sigbuilder block){tuvar=[0:10]}
      mask help: Simulink:masks:SigbuilderBlock_MD
      mask init:
      | if ~strcmp(get_param(bdroot(gcbh),'SimulationStatus'),'stopped') tuvar = sigbuilder_block('maskInit'); end
      settings: CopyFcn=sigbuilder_block('copy');  DeleteFcn=sigbuilder_block('delete');  ModelCloseFcn=sigbuilder_block('modelClose');  PreSaveFcn=sigbuilder_block('preSave');  PauseFcn=sigbuilder_block('pause');  ContinueFcn=sigbuilder_block('continue');  NameChangeFcn=sigbuilder_block('namechange');  OpenFcn=sigbuilder_block('open',[437.25 153 550.5 359.25 ]);  CloseFcn=sigbuilder_block('close');
      mask Display: plot(0, 0, 100, 100,[2, 2, 32, 32, 2], [68, 8, 8, 68, 68],[32, 2], [38, 38], [32, 19, 2],[53, 60, 44], [32, 17, 17, 2],[16, 16, 31, 31]);txt = getActiveGroup(gcbh);text(2, 100, txt,'verticalAlignment', 'top');
  Sum2 : Sum  Inputs=|++
  Switch : Switch  Criteria=u2 > Threshold  Threshold=2
  Transfer Fcn2 : TransferFcn  Denominator=[0.25e-06 0 1]
  Transfer Fcn3 : TransferFcn  Numerator=[-25e-03 0]  Denominator=[0.25e-06 0 1]
  Vout : Outport
  Iout : Outport  Port=2
  wires:
  Transfer Fcn3/1 -> Sum2/2
  Vin/1 -> Transfer Fcn2/1
  Transfer Fcn2/1 -> Sum2/1
  Sum2/1 -> Vout/1, Gain1/1, Gain3/1
  Signal Builder/1(Signal 1) -> Switch/2
  Gain1/1 -> Switch/1
  Gain3/1 -> Iout/1, Transfer Fcn3/1

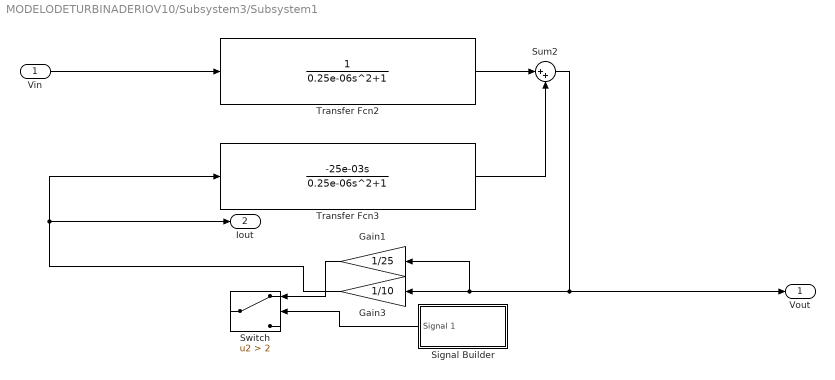
== system MODELODETURBINADERIOV10/Subsystem3/Subsystem1 ==
  Vin : Inport
  Gain1 : Gain  Gain=1/25
  Gain3 : Gain  Gain=1/10
  Signal Builder : Subsystem  Tag=STV Subsys  LoadFcn=sigbuilder_block('load');  StartFcn=sigbuilder_block('start');  StopFcn=sigbuilder_block('stop');  ClipboardFcn=sigbuilder_block('clipboard');  mask(Sigbuilder block){tuvar=[0:10]}
      mask help: Simulink:masks:SigbuilderBlock_MD
      mask init:
      | if ~strcmp(get_param(bdroot(gcbh),'SimulationStatus'),'stopped') tuvar = sigbuilder_block('maskInit'); end
      settings: CopyFcn=sigbuilder_block('copy');  DeleteFcn=sigbuilder_block('delete');  ModelCloseFcn=sigbuilder_block('modelClose');  PreSaveFcn=sigbuilder_block('preSave');  PauseFcn=sigbuilder_block('pause');  ContinueFcn=sigbuilder_block('continue');  NameChangeFcn=sigbuilder_block('namechange');  OpenFcn=sigbuilder_block('open',[437.25 153 550.5 359.25 ]);  CloseFcn=sigbuilder_block('close');
      mask Display: plot(0, 0, 100, 100,[2, 2, 32, 32, 2], [68, 8, 8, 68, 68],[32, 2], [38, 38], [32, 19, 2],[53, 60, 44], [32, 17, 17, 2],[16, 16, 31, 31]);txt = getActiveGroup(gcbh);text(2, 100, txt,'verticalAlignment', 'top');
  Sum2 : Sum  Inputs=|++
  Switch : Switch  Criteria=u2 > Threshold  Threshold=2
  Transfer Fcn2 : TransferFcn  Denominator=[0.25e-06 0 1]
  Transfer Fcn3 : TransferFcn  Numerator=[-25e-03 0]  Denominator=[0.25e-06 0 1]
  Vout : Outport
  Iout : Outport  Port=2
  wires:
  Transfer Fcn2/1 -> Sum2/1
  Vin/1 -> Transfer Fcn2/1
  Transfer Fcn3/1 -> Sum2/2
  Sum2/1 -> Gain1/1, Gain3/1, Vout/1
  Signal Builder/1(Signal 1) -> Switch/2
  Gain1/1 -> Switch/1
  Gain3/1 -> Iout/1, Transfer Fcn3/1

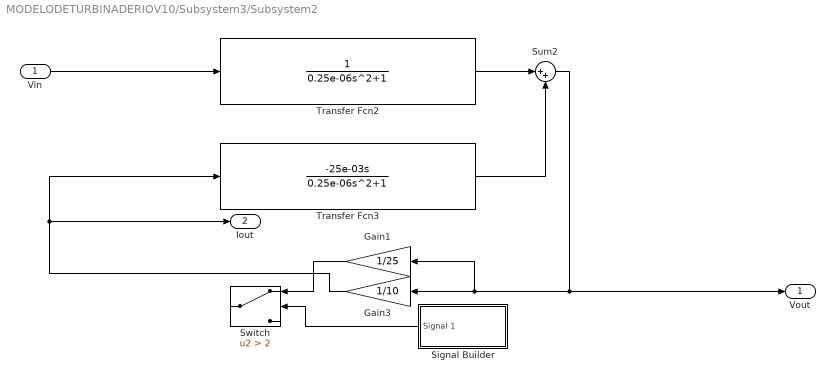
== system MODELODETURBINADERIOV10/Subsystem3/Subsystem2 ==
  Vin : Inport
  Gain1 : Gain  Gain=1/25
  Gain3 : Gain  Gain=1/10
  Signal Builder : Subsystem  Tag=STV Subsys  LoadFcn=sigbuilder_block('load');  StartFcn=sigbuilder_block('start');  StopFcn=sigbuilder_block('stop');  ClipboardFcn=sigbuilder_block('clipboard');  mask(Sigbuilder block){tuvar=[0:10]}
      mask help: Simulink:masks:SigbuilderBlock_MD
      mask init:
      | if ~strcmp(get_param(bdroot(gcbh),'SimulationStatus'),'stopped') tuvar = sigbuilder_block('maskInit'); end
      settings: CopyFcn=sigbuilder_block('copy');  DeleteFcn=sigbuilder_block('delete');  ModelCloseFcn=sigbuilder_block('modelClose');  PreSaveFcn=sigbuilder_block('preSave');  PauseFcn=sigbuilder_block('pause');  ContinueFcn=sigbuilder_block('continue');  NameChangeFcn=sigbuilder_block('namechange');  OpenFcn=sigbuilder_block('open',[437.25 153 550.5 359.25 ]);  CloseFcn=sigbuilder_block('close');
      mask Display: plot(0, 0, 100, 100,[2, 2, 32, 32, 2], [68, 8, 8, 68, 68],[32, 2], [38, 38], [32, 19, 2],[53, 60, 44], [32, 17, 17, 2],[16, 16, 31, 31]);txt = getActiveGroup(gcbh);text(2, 100, txt,'verticalAlignment', 'top');
  Sum2 : Sum  Inputs=|++
  Switch : Switch  Criteria=u2 > Threshold  Threshold=2
  Transfer Fcn2 : TransferFcn  Denominator=[0.25e-06 0 1]
  Transfer Fcn3 : TransferFcn  Numerator=[-25e-03 0]  Denominator=[0.25e-06 0 1]
  Vout : Outport
  Iout : Outport  Port=2
  wires:
  Transfer Fcn3/1 -> Sum2/2
  Vin/1 -> Transfer Fcn2/1
  Transfer Fcn2/1 -> Sum2/1
  Sum2/1 -> Vout/1, Gain1/1, Gain3/1
  Signal Builder/1(Signal 1) -> Switch/2
  Gain1/1 -> Switch/1
  Gain3/1 -> Iout/1, Transfer Fcn3/1

== system MODELODETURBINADERIOV10/Subsystem3/abc2dq1 ==
  abc : Inport
  sin cos : Inport  Port=2
  Demux2 : Demux  Outputs=3
  Terminator : Terminator
  abc_to_dq0 Transformation : powerlib_extras/Measurements/abc_to_dq0 Transformation
  d : Outport
  q : Outport  Port=2
  wires:
  sin cos/1 -> abc_to_dq0 Transformation/2
  abc/1 -> abc_to_dq0 Transformation/1
  abc_to_dq0 Transformation/1 -> Demux2/1
  Demux2/2 -> q/1
  Demux2/1 -> d/1
  Demux2/3 -> Terminator/1

== system MODELODETURBINADERIOV10/Subsystem3/abc2dq2 ==
  abc : Inport
  sin cos : Inport  Port=2
  Demux2 : Demux  Outputs=3
  Terminator : Terminator
  abc_to_dq0 Transformation : powerlib_extras/Measurements/abc_to_dq0 Transformation
  d : Outport
  q : Outport  Port=2
  wires:
  Demux2/3 -> Terminator/1
  Demux2/1 -> d/1
  Demux2/2 -> q/1
  abc_to_dq0 Transformation/1 -> Demux2/1
  abc/1 -> abc_to_dq0 Transformation/1
  sin cos/1 -> abc_to_dq0 Transformation/2

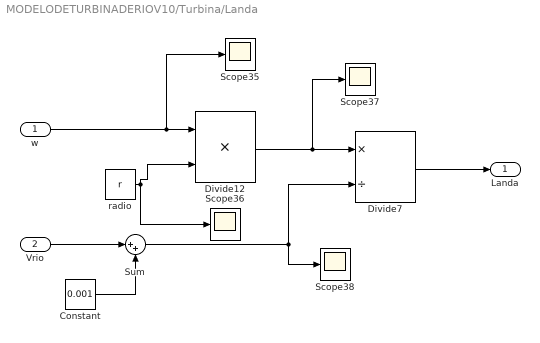
== system MODELODETURBINADERIOV10/Turbina/Landa ==
  w : Inport
  Vrio : Inport  Port=2
  Constant : Constant  Value=0.001
  Divide12 : Product  Inputs=**
  Divide7 : Product  Inputs=*/
  Scope{35..38} (4 alike) : Scope
  Sum : Sum  Inputs=|++
  radio : Constant  Value=r
  Landa : Outport
  wires:
  Divide7/1 -> Landa/1
  radio/1 -> Divide12/2, Scope36/1
  Divide12/1 -> Scope37/1, Divide7/1
  w/1 -> Scope35/1, Divide12/1
  Vrio/1 -> Sum/1
  Sum/1 -> Scope38/1, Divide7/2
  Constant/1 -> Sum/2

== system MODELODETURBINADERIOV10/Turbina/Landai ==
  Beta : Inport
  Landa : Inport  Port=2
  lamdai : MATLAB Function  TreatAsAtomicUnit=on
  Landai : Outport
  wires:
  lamdai/1(Ii) -> Landai/1
  Landa/1 -> lamdai/2(landa)
  Beta/1 -> lamdai/1(beta)

== system MODELODETURBINADERIOV10/Turbina/Modelo2 ==
  Cp : Inport
  Vrio : Inport  Port=2
  A1 : Constant  Value=A
  Constant4 : Constant  Value=3
  D1 : Constant  Value=den
  Divide13 : Product  Inputs=****  SaturateOnIntegerOverflow=on  RndMeth=Zero
  Gain11 : Gain  Gain=0.5
  Math Function6 : Math  Operator=pow  SaturateOnIntegerOverflow=on
  Pm : Outport
  wires:
  Constant4/1 -> Math Function6/2
  Divide13/1 -> Gain11/1
  D1/1 -> Divide13/3
  Cp/1 -> Divide13/1
  Gain11/1 -> Pm/1
  A1/1 -> Divide13/2
  Vrio/1 -> Math Function6/1
  Math Function6/1 -> Divide13/4

== system MODELODETURBINADERIOV10/Subsystem3/Subsystem/Signal Builder ==
  Demux : Demux  Tag=STV Demux  Outputs=1
  FromWs : FromWorkspace  Tag=STV FromWs  VariableName=tuvar  SampleTime=0
      SigBuilderData=|
      | common.afterFinalStr = 'Extrapolate'
      | common.sampleTime = 0
      | dataSet.timeRange = [0 1]
      | dataSet.name = 'Group 1'
      | sbobj.Groups.Name = 'Group 1'
      | sbobj.Groups.Signals.Name = 'Signal 1'
      | sbobj.Groups.Signals.XData = [0 0.102 0.102 0.3 0.3 1]
      | sbobj.Groups.Signals.YData = [0 0 3 3 0 0]
      | sbobj.Groups.TimeRange = [0 1]
  Signal 1 : Outport  Tag=STV Outport
  wires:
  Demux/1 -> Signal 1/1
  FromWs/1 -> Demux/1

== system MODELODETURBINADERIOV10/Subsystem3/Subsystem1/Signal Builder ==
  Demux : Demux  Tag=STV Demux  Outputs=1
  FromWs : FromWorkspace  Tag=STV FromWs  VariableName=tuvar  SampleTime=0
      SigBuilderData=|
      | common.afterFinalStr = 'Extrapolate'
      | common.sampleTime = 0
      | dataSet.timeRange = [0 1]
      | dataSet.name = 'Group 1'
      | sbobj.Groups.Name = 'Group 1'
      | sbobj.Groups.Signals.Name = 'Signal 1'
      | sbobj.Groups.Signals.XData = [0 0.102 0.102 0.3 0.3 1]
      | sbobj.Groups.Signals.YData = [0 0 3 3 0 0]
      | sbobj.Groups.TimeRange = [0 1]
  Signal 1 : Outport  Tag=STV Outport
  wires:
  Demux/1 -> Signal 1/1
  FromWs/1 -> Demux/1

== system MODELODETURBINADERIOV10/Subsystem3/Subsystem2/Signal Builder ==
  Demux : Demux  Tag=STV Demux  Outputs=1
  FromWs : FromWorkspace  Tag=STV FromWs  VariableName=tuvar  SampleTime=0
      SigBuilderData=|
      | common.afterFinalStr = 'Extrapolate'
      | common.sampleTime = 0
      | dataSet.timeRange = [0 1]
      | dataSet.name = 'Group 1'
      | sbobj.Groups.Name = 'Group 1'
      | sbobj.Groups.Signals.Name = 'Signal 1'
      | sbobj.Groups.Signals.XData = [0 0.102 0.102 0.3 0.3 1]
      | sbobj.Groups.Signals.YData = [0 0 3 3 0 0]
      | sbobj.Groups.TimeRange = [0 1]
  Signal 1 : Outport  Tag=STV Outport
  wires:
  Demux/1 -> Signal 1/1
  FromWs/1 -> Demux/1

== matlab function MODELODETURBINADERIOV10/Turbina/MATLAB Function3 ==
  data: beta input; y output; landa input; Ii input
function y = fcn(beta, landa,Ii)
w=0.5176; 
w1=116/Ii;
 w2=0.4*beta;
 w3=exp(-21/Ii);
 
 cp=w*(w1-w2-5)*w3+0.0068*landa;
 
 
 
 
 
y=cp;

== matlab function MODELODETURBINADERIOV10/Turbina/Landai/lamdai ==
  data: beta input; Ii output; landa input
function Ii = fcn(beta,landa)


Iii=(1/((landa+(0.08*beta))))-((0.035)/((beta^3)+1));
Ii=1/Iii;
